simulink model "larix2_tuner_openLoop"  (R2020b)
settings: Solver=FixedStepDiscrete  StartTime=0.0  StopTime=6  FixedStep=0.002  RelTol=1e-3
PostLoadFcn:
  | load('ThrustTable.mat');
  | init();
values from neighbouring files (symbols this model uses):
  eul_0 = [-45*pi/180 0 0]    [init.m]
  g = 9.810    (= 9.81)    [init.m]
  omega_0 = [0 0 0]    [init.m]
  pos_0 = [0 0 0]    [init.m]
  vel_0 = [0 0 0]    [init.m]
undefined symbols (not defined in the file or in its folder): DiscIntNeverNeededParam
libraries: sharedtransform x2
settings Model: Creator=ac114611  LastModifiedBy=wendelin
settings DataIOCC: ExternalInput=getinputstruct(spec2)  InitialState=getstatestruct(spec2)  ReturnWorkspaceOutputs=off
settings OptimizationCC: DefaultParameterBehavior=Inlined  EnhancedBackFolding=on  PassReuseOutputArgsAs=Individual arguments  MaxStackSize=64  OptimizeBlockOrder=speed  DifferentSizesBufferReuse=on  EfficientTunableParamExpr=on
settings DebuggingCC: ParameterPrecisionLossMsg=none  ParameterTunabilityLossMsg=error  ArithmeticOperatorsInVariantConditions=warning
settings HardwareCC: ProdBitPerPointer=32  ProdBitPerSizeT=32  ProdBitPerPtrDiffT=32  ProdLargestAtomicInteger=Long  ProdLargestAtomicFloat=Double  ProdWordSize=32  ProdHWDeviceType=ARM Compatible->ARM Cortex  TargetBitPerLong=64  TargetBitPerPointer=64  TargetBitPerSizeT=64  TargetBitPerPtrDiffT=64  TargetLongLongMode=on  TargetIntDivRoundTo=Zero  TargetEndianess=LittleEndian  TargetWordSize=64  TargetHWDeviceType=MATLAB Host  ProdEqTarget=off
settings SFSimCC: SimUseLocalCustomCode=off  MATLABDynamicMemAlloc=off  CustomCodeUndefinedFunction=UseInterfaceOnly
settings RTWCC: Description=Embedded Coder  SystemTargetFile=ert.tlc  GenCodeOnly=on  PackageName=larix2_codegen.zip  TemplateMakefile=ert_default_tmf  RTWUseLocalCustomCode=off  Toolchain=GNU gcc/g++ | gmake (64-bit Linux)  IncludeHyperlinkInReport=on  GenerateCodeMetricsReport=on
settings CodeAppCC: ForceParamTrailComments=on  IgnoreCustomStorageClasses=off  OperatorAnnotations=on  SimulinkDataObjDesc=on  SFDataObjDesc=on  InsertBlockDesc=on
settings ERTTargetCC: TargetLangStandard=C99 (ISO)  InlinedParameterPlacement=NonHierarchical  ERTCustomFileTemplate=example_file_process.tlc

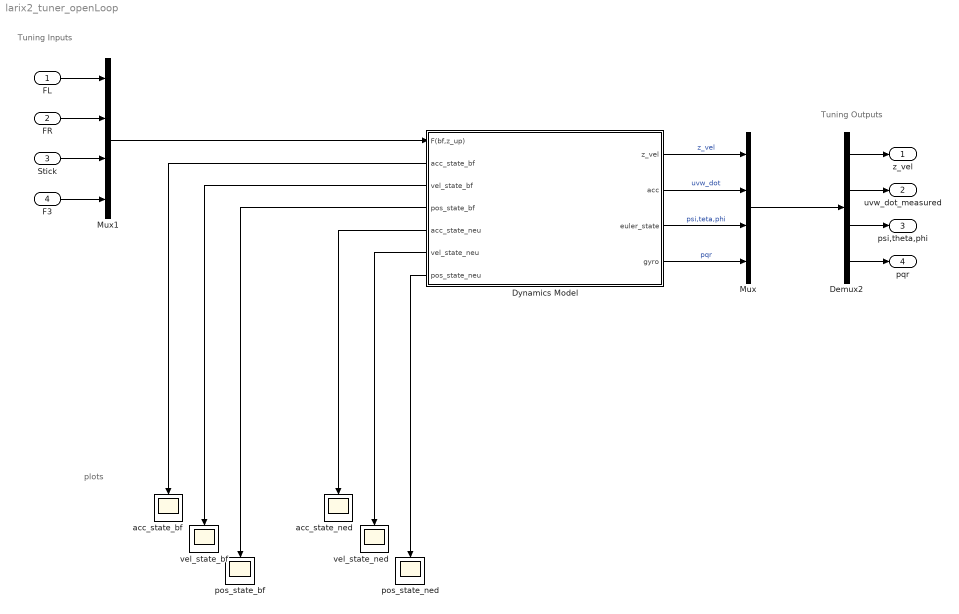
== system larix2_tuner_openLoop ==
  note: Tuning Inputs
  note: Tuning Outputs
  note: plots
  FL : Inport  PortDimensions=1
  FR : Inport  Port=2
  Stick : Inport  Port=3
  F3 : Inport  Port=4
  Demux2 : Demux
  Dynamics Model : Subsystem
      settings: PortSchema="{\"entries\":[{\"content\":{\"sides\":[{\"content\":{\"connectorIds\":[\"In1\",\"Out5\",\"Out6\",\"Out7\",\"Out8\",\"Out9\",\"Out10\"]},\"type\":\"ConnectorPlacement.EquallySpacedRectSide\",\"uuid\":\"7b482eda-451f-4705-a72e-674db1e2ea8f\"},{\"content\":{\"connectorIds\":[\"Out1\",\"Out2\",\"Out3\",\"Out4\"],\"side\":\"RIGHT\"},\"type\":\"ConnectorPlacement.EquallySpacedRectSide\",\"uuid\":\"2344d3e9-2a2c-4bd3-8790-1f9d37abcd4c\"},{\"content\":{\"connectorIds\":[],\"side\":\"TOP\"},\"type\":\"ConnectorPlacement.EquallySpacedRectSide\",\"uuid\":\"13a22bb4-0a82-4477-a366-02f381e5ef07\"},{\"content\":{\"connectorIds\":[],\"side\":\"BOTTOM\"},\"type\":\"ConnectorPlacement.EquallySpacedRectSide\",\"uuid\":\"663825dc-fe4c-484f-87e0-eae3c1c76089\"},{\"content\":{\"connectorIds\":[],\"side\":\"HIDDEN\"},\"type\":\"ConnectorPlacement.EquallySpacedRectSide\",\"uuid\":\"0874c0d1-0ac2-489a-adcf-241d9ac40396\"}]},\"type\":\"ConnectorPlacement.EquallySpacedConnector\",\"uuid\":\"4f633129-49ae-43ab-aa97-bf1abe451306\"}],\"packageUris\":[\"http://schema.mathworks.com/mf0/Connector/R2020b\"],\"version\":\"1.0\"}"
  Mux : Mux
  Mux1 : Mux
  acc_state_bf : Scope
  acc_state_ned : Scope
  pos_state_bf : Scope
  pos_state_ned : Scope
  vel_state_bf : Scope
  vel_state_ned : Scope
  z_vel : Outport  PortDimensions=1
  uvw_dot_measured : Outport  Port=2  PortDimensions=3
  psi,theta,phi : Outport  Port=3  PortDimensions=3
  pqr : Outport  Port=4  PortDimensions=3
  wires:
  Dynamics Model/4(gyro) -> Mux/4  "pqr"
  Dynamics Model/2(acc) -> Mux/2  "uvw_dot"
  Dynamics Model/1(z_vel) -> Mux/1  "z_vel"
  Dynamics Model/3(euler_state) -> Mux/3  "psi,teta,phi"
  Mux/1 -> Demux2/1
  Demux2/1 -> z_vel/1
  Demux2/2 -> uvw_dot_measured/1
  Demux2/4 -> pqr/1
  Demux2/3 -> psi,theta,phi/1
  FL/1 -> Mux1/1
  FR/1 -> Mux1/2
  Stick/1 -> Mux1/3
  F3/1 -> Mux1/4
  Dynamics Model/8(acc_state_neu) -> acc_state_ned/1
  Dynamics Model/6(vel_state_bf) -> vel_state_bf/1
  Dynamics Model/9(vel_state_neu) -> vel_state_ned/1
  Dynamics Model/5(acc_state_bf) -> acc_state_bf/1
  Dynamics Model/7(pos_state_bf) -> pos_state_bf/1
  Dynamics Model/10(pos_state_neu) -> pos_state_ned/1
  Mux1/1 -> Dynamics Model/1(F(bf,z_up))

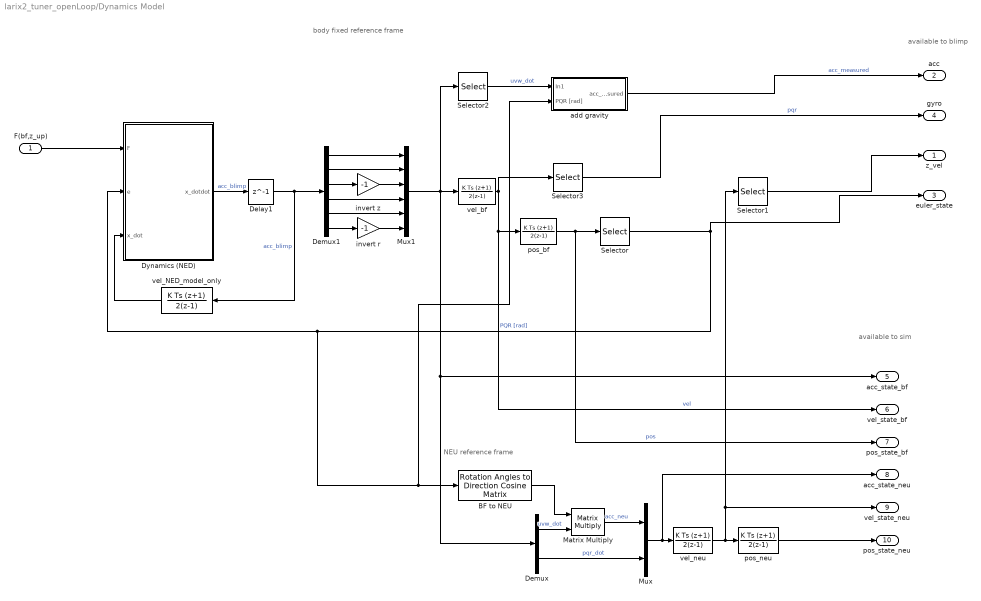
== system larix2_tuner_openLoop/Dynamics Model ==
  note: NEU reference frame
  note: body fixed reference frame
  note: available
      | to sim
  note: available
      | to blimp
  F(bf,z_up) : Inport
  " BF to NEU" : sharedtransform/Rotation Angles to Direction Cosine Matrix  rotationOrder=XYZ  aMode=aMode
      settings: SourceProductBaseCode=AE,PW,MT,UV,VE,VP
  Delay1 : Delay  DelayLength=1  StateName=acc_NED_delay
  Demux : Demux  Outputs=2
  Demux1 : Demux  Outputs=6
  Dynamics (NED) : MATLAB Function  TreatAsAtomicUnit=on
  Matrix Multiply : Product  Multiplication=Matrix(*)
  Mux : Mux  Inputs=2
  Mux1 : Mux  Inputs=6
  Selector : Selector  InputPortWidth=6  IndexOptions=Index vector (dialog)  Indices=[4 5 6]  OutputSizes=1
  Selector1 : Selector  InputPortWidth=6  IndexOptions=Index vector (dialog)  Indices=[3]  OutputSizes=1
  Selector2 : Selector  InputPortWidth=6  IndexOptions=Index vector (dialog)  Indices=[1 2 3]  OutputSizes=1
  Selector3 : Selector  InputPortWidth=6  IndexOptions=Index vector (dialog)  Indices=[4 5 6]  OutputSizes=1
  add gravity : Subsystem
  invert r : Gain  Gain=-1
  invert z : Gain  Gain=-1
  pos_bf : DiscreteIntegrator  IntegratorMethod=Integration: Trapezoidal  InitialCondition=[pos_0,eul_0]  SampleTime=-1  StateName=position_bf  ICPrevOutput=DiscIntNeverNeededParam  ICPrevScaledInput=DiscIntNeverNeededParam
  pos_neu : DiscreteIntegrator  IntegratorMethod=Integration: Trapezoidal  InitialCondition=[pos_0';eul_0']  SampleTime=-1  StateName=position_neu  ICPrevOutput=DiscIntNeverNeededParam  ICPrevScaledInput=DiscIntNeverNeededParam
  vel_NED_model_only : DiscreteIntegrator  IntegratorMethod=Integration: Trapezoidal  SampleTime=-1  StateName=vel_ned  ICPrevOutput=DiscIntNeverNeededParam  ICPrevScaledInput=DiscIntNeverNeededParam
  vel_bf : DiscreteIntegrator  IntegratorMethod=Integration: Trapezoidal  InitialCondition=[vel_0,omega_0]  SampleTime=-1  StateName=velocity_bf  ICPrevOutput=DiscIntNeverNeededParam  ICPrevScaledInput=DiscIntNeverNeededParam
  vel_neu : DiscreteIntegrator  IntegratorMethod=Integration: Trapezoidal  InitialCondition=[pos_0';eul_0']  SampleTime=-1  StateName=velocity_neu  ICPrevOutput=DiscIntNeverNeededParam  ICPrevScaledInput=DiscIntNeverNeededParam
  z_vel : Outport  OutDataTypeStr=double
  acc : Outport  Port=2  OutDataTypeStr=double
  euler_state : Outport  Port=3  OutDataTypeStr=double
  gyro : Outport  Port=4  OutDataTypeStr=double
  acc_state_bf : Outport  Port=5
  vel_state_bf : Outport  Port=6  OutDataTypeStr=double
  pos_state_bf : Outport  Port=7
  acc_state_neu : Outport  Port=8
  vel_state_neu : Outport  Port=9
  pos_state_neu : Outport  Port=10
  wires:
  pos_bf/1 -> pos_state_bf/1, Selector/1  "pos"
  vel_bf/1 -> pos_bf/1, vel_state_bf/1, Selector3/1  "vel"
  F(bf,z_up)/1 -> Dynamics (NED)/1(F)
  Dynamics (NED)/1(x_dotdot) -> Delay1/1  "acc_blimp"
  Selector3/1 -> gyro/1  "pqr"
  pos_neu/1 -> pos_state_neu/1
  Demux/1 -> Matrix Multiply/2  "uvw_dot"
  Demux/2 -> Mux/2  "pqr_dot"
  Matrix Multiply/1 -> Mux/1  "acc_neu"
  Selector/1 -> add gravity/2(PQR [rad]), " BF to NEU"/1, Dynamics (NED)/2(e), euler_state/1  "PQR [rad]"
  " BF to NEU"/1 -> Matrix Multiply/1
  Selector2/1 -> add gravity/1(In1)  "uvw_dot"
  Mux/1 -> acc_state_neu/1, vel_neu/1
  vel_neu/1 -> Selector1/1, vel_state_neu/1, pos_neu/1
  Delay1/1 -> vel_NED_model_only/1, Demux1/1  "acc_blimp"
  Mux1/1 -> Selector2/1, acc_state_bf/1, Demux/1, vel_bf/1
  vel_NED_model_only/1 -> Dynamics (NED)/3(x_dot)
  Demux1/1 -> Mux1/1
  Demux1/2 -> Mux1/2
  Demux1/3 -> invert z/1
  invert z/1 -> Mux1/3
  Demux1/4 -> Mux1/4
  Demux1/5 -> Mux1/5
  Demux1/6 -> invert r/1
  invert r/1 -> Mux1/6
  Selector1/1 -> z_vel/1
  add gravity/1(acc_bf_measured) -> acc/1  "acc_measured"

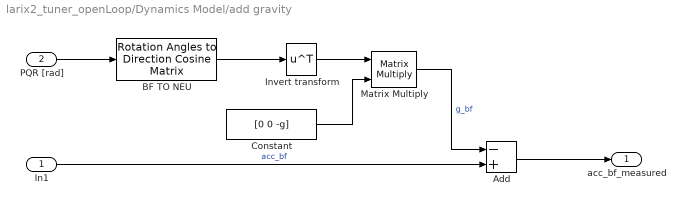
== system larix2_tuner_openLoop/Dynamics Model/add gravity ==
  In1 : Inport
  PQR [rad] : Inport  Port=2
  Add : Sum  Inputs=-+
  BF TO NEU : sharedtransform/Rotation Angles to Direction Cosine Matrix  rotationOrder=XYZ  aMode=aMode
      settings: SourceProductBaseCode=AE,PW,MT,UV,VE,VP
  Constant : Constant  Value=[0 0 -g]
  Invert transform : Math  Operator=transpose  SaturateOnIntegerOverflow=on
  Matrix Multiply : Product  Multiplication=Matrix(*)
  acc_bf_measured : Outport
  wires:
  In1/1 -> Add/2  "acc_bf"
  BF TO NEU/1 -> Invert transform/1
  PQR [rad]/1 -> BF TO NEU/1
  Invert transform/1 -> Matrix Multiply/1
  Matrix Multiply/1 -> Add/1  "g_bf"
  Constant/1 -> Matrix Multiply/2
  Add/1 -> acc_bf_measured/1

== matlab function larix2_tuner_openLoop/Dynamics Model/Dynamics (NED) ==
  data: F input; x_dotdot output; e input; x_dot input
function x_dotdot = fcn(F,e,x_dot)

fL = F(1);
fR = F(2);
stick = F(3);
fB = F(4);

roll = e(1);
pitch = e(2);
yaw = e(3);
%e3 = e(4);


u = x_dot(1);
v = x_dot(2);
w = x_dot(3);
p = x_dot(4);
q = x_dot(5);
r = x_dot(6);

%}

g = 9.81;
rho_air = 1.225; 
eta_air = 1.802e-5;



blimp = inertias();
prp = blimp.prp;
par = blimp.par;
in = blimp.mM;




mx = in.M(1,1);
my = in.M(2,2);
mz = in.M(3,3);

Jxx = in.M(4,4);
Jyy = in.M(5,5);
Jzz = in.M(6,6);
Jxz = in.M(3,6);
 
%DYNAMICS

f1 = -mz*w*q + my*r*v + in.mass*(in.a(1)*( q^2 + r^2) - in.a(3)*r*p);
f2 = -mx*u*r + mz*p*w + in.mass*(-in.a(1)*p*q - in.a(3)*r*q);
f3 = -my*v*p + mx*q*u + in.mass*(-in.a(1)*r*p + in.a(3)*(q^2 + p^2));
f4 = -(Jzz - Jyy)*r*q + Jxz*p*q + in.mass*in.a(3)*(u*r - p*w);
f5 = -(Jxx - Jzz)*p*r + Jxz*(r^2 - p^2) + in.mass*(in.a(1)*(v*p - q*u) - in.a(3)*(w*q - r*v));
f6 = -(Jyy - Jxx)*q*p - Jxz*q*r + in.mass*(-in.a(1)*(u*r - p*w));


F = [f1; f2; f3; f4; f5; f6];

%GRAVITATIONAL FORCES Quaternion
%{
DCM = [e0^2+e1^2-e2^2-e3^2, 2*(e1*e2-e0*e3),2*(e0*e2-e1*e3);...
        2*(e0*e3-e1*e2),e0^2-e1^2+e2^2-e3^2,2*(e2*e3-e0*e1);...
        2*(e1*e3-e0*e2),2*(e0*e1-e2*e3),e0^2-e1^2-e2^2+e3^2];


    
G = [DCM(3,1)*(W+B); DCM(3,2)*(W+B); DCM(3,3)*(W+B);DCM(3,2)*in.a(3)*W; (DCM(3,1)*in.a(3)-DCM(3,3)*in.a(1))*W; DCM(3,2)*in.a(1)*W];
%}



%GRAVITATIONAL FORCES EULER
%{
g_vec = [0 0 g]';

%rot = eul2rotm([e0 e1 e2],'XYZ')';
rot = eul2rotm([roll pitch yaw],'XYZ')';

G_forces = [0 0 h]'*rot*g_vec;

gondola_mass = par.gondola_body.mass + par.gondola_support.mass + par.stick.mass + 2*par.blade_left.mass;      %mass of the whole gondola assembly with its CG at [CG_stick_x 0 CG_stick_z]

G_gondola = gondola_mass*rot*g_vec;


CG_ga = par.stick.position';    %CG coordinates from CV to Gondola assembly

G_moments = cross(G_gondola, CG_ga);

G = [G_forces; G_moments];
%}

h = prp.mass_H;
B = prp.volume_blimp_body*prp.density_air*g;
W = B + h*g;
%%{
rot = eul2rotm([roll pitch yaw],'XYZ');

G = [rot(3,1)*(W-B), rot(3,2)*(W-B), rot(3,3)*(W-B), -rot(3,2)*in.CG(3)*W, (rot(3,1)*in.CG(3) - rot(3,3)*in.CG(1))*W, rot(3,2)*in.CG(1)*W]';
%}
%{
g_vec = [0 0 g];

rotNEDtoBF = eul2rotm([roll pitch yaw],'XYZ');

g_bf = g_vec*rotNEDtoBF;

G = [h*g_bf, cross(in.CG,W*g_bf)]';
%}


%PROPULSION FORCES


rL = blimp.par.blade_left.position';
rR = blimp.par.blade_right.position';
rB = blimp.par.bot_rud_motor.position';

FL = fL*[sin(-stick*pi/2) 0 cos(-stick*pi/2)]';
FR = fR*[sin(-stick*pi/2) 0 cos(-stick*pi/2)]';
FB = fB*[0 1 0]';

TL = cross(rL,FL);
TR = cross(rR,FR);
TB = cross(rB,FB);

Forces = FL+FR+FB;
Torques = TL+TR+TB;

P_NED = [Forces;Torques];

P = P_NED.*[1 1 -1 1 1 -1]';        %convert P from NEU (allocation) to NED 


% AERO FORCES

%AR ~= 0.7 --> nu_fin (Modeling and Simulation of Airship Dynamics)
%finenessratio = 2.375
%hull projected area = 7.461m^2   effective fin area = 0.64 m^2
% effective fin area/ hull projected area = 0.086 --> nu hull

nu_hull =  1.01;
nu_fin = 0.58;

%Cdh0 = 0.3;     %from summary of drag coefficients of various shaped cylinders but reduced because ellipsoid    
Cdh0 = 0.07;    %Theory and Practice of the Hydrodynamic Redesign of Artificial Hellbender Habitat --> closer to value from other papers
Cdf0 = 0.007;    %from Hoerner SF. Fluid Dynamic Drag, Hoerner Fluid Dynamics, 1965. 
Cdg0 = 0.5;     %from Hoerner SF. Fluid Dynamic Drag, Hoerner Fluid Dynamics, 1965. 

Cdhc = 0.5;
Cdfc = 1.2;     %from Hoerner SF. Fluid Dynamic Drag, Hoerner Fluid Dynamics, 1965. 
Cdgc = 0.8;

e = sqrt((prp.length_blimp_a1^2 + prp.radius_blimp_body^2)/prp.length_blimp_a1);

S = pi*prp.radius_blimp_body*(prp.radius_blimp_body+(prp.length_blimp_a1^2)*sin(e)/e);

Vh_ref = prp.volume_blimp_body; %volume based on two semi ellipsoids
Sg_ref = prp.volume_gondola_body^(2/3);
Sh_ref = S;
Sf_ref = 2*prp.surface_two_fins;


fh = (prp.length_tip_to_fin - prp.length_blimp_a1)/prp.length_blimp_a2;
xcv = prp.length_blimp_a1+(3/8)*(prp.length_blimp_a2-prp.length_blimp_a1);
%xcv = prp.length_blimp_a1 - (4*pi/3)*(prp.length_blimp_a1-prp.length_blimp_a2);

I_1 = pi*((prp.radius_blimp_body^2)/Sh_ref)*(1-fh^2);
I_3 = pi*((prp.radius_blimp_body^2)/(3*prp.length_blimp_body*Sh_ref)*(prp.length_blimp_a1 - 2*prp.length_blimp_a2*(fh^3) - 3*prp.length_blimp_a1*(fh^2)) - xcv*I_1/prp.length_blimp_body);


J_1 = prp.radius_blimp_body/(2*Sh_ref)*(pi*prp.length_blimp_a1 + prp.length_blimp_a2*sqrt(1-fh^2)*fh + 2*prp.length_blimp_a2*asin(fh));
J_2 = (J_1/prp.length_blimp_body)*(prp.length_blimp_a1-xcv) + (2*prp.radius_blimp_body/(3*prp.length_blimp_body*Sh_ref))*(prp.length_blimp_a2^2 - prp.length_blimp_a1^2 - (prp.length_blimp_a2^2)*(1-fh^2)^(3/2));

%{
if u == 0
    Cf = 0;
else
Re = abs(u)*prp.length_blimp_body*rho_air/eta_air;
Cf = 0.045*Re^(-1/6);
end

%Cdchull = 1.17;     %Cd of cylinder in transverse flow
%Cdcfin = 1.28;       %Cd of Plate in transverse flow

%Cdcross = -(1/S_ref)*(Cdchull*J_1*S_ref+Cdcfin*S_fin);
%lf1 = 2.35;          %origin to aero/geo center of fin
%lf2 = 2.5;
%}




lf1 = prp.length_tip_to_ac_fin;            %tip to aero center of fin
lf2 = prp.length_tip_to_gc_fin;              %tip to geo center of fin
lf3 = prp.length_yz_origin_to_ac_fin;

U_abs = sqrt(u^2 +v^2 +w^2);


a = atan2(w,u);

if a < 0
    LS = -liftslope(-a);
else
    LS = liftslope(a);
end
    


if U_abs == 0
    b = 0;
else
    b = asin(v/U_abs);
end


%Cx1 = -Cf*(4*(prp.length_blimp_body/prp.radius_blimp_body)^(1/3)+6*(prp.length_blimp_body/prp.radius_blimp_body)^(-1.2)+24*(prp.length_blimp_body/prp.radius_blimp_body)^(-2.7)); %Cd0H        KTh paper       cgcl_xial Cd & b as mcgcl_x_diameter/2 
Cx1 = -(Cdh0*Sh_ref + Cdf0*Sf_ref + Cdg0*Sg_ref);
Cx2 = (in.k(2)-in.k(1))*nu_hull*I_1*Sh_ref;             %munk lift
Cx3 = 0;

Cy1 = -Cx2;                                       
Cy2 = -0.5*LS*Sf_ref*nu_fin;                               %dCl/da = 2*pi  --> only for small angle of attack     from On the lift curve slope for rectangular flat plate wings at moderate Reynolds number
Cy3 = -(Cdhc*J_1*Sh_ref+Cdfc*Sf_ref + Cdgc*Sg_ref);
Cy4 = 0;

Cz1 = -Cx2;
Cz2 = Cy2;
Cz3 = -(Cdhc*J_1*Sh_ref + Cdfc*Sf_ref);       
Cz4 = Cy4;

Cl1 = 0;
Cl2 = Cdgc*Sg_ref*par.gondola_body.position(3);
Cl3 = Cdgc*Sg_ref*par.gondola_body.position(3)*prp.length_blimp_body^2;
Cl4 = -(Cdgc*Sg_ref*par.gondola_body.position(3) + Cdfc*Sf_ref*lf3)*(2*prp.radius_blimp_body)^2;

Cm1 = -(in.k(2)-in.k(1))*nu_hull*I_3*Sh_ref*prp.length_blimp_body;
Cm2 = -0.5*LS*Sf_ref*nu_fin*lf1;
Cm3 = -(Cdhc*J_2*Sh_ref*prp.length_blimp_body + Cdfc*Sf_ref*lf2);
Cm4 = 0;
Cm5 = -Cdfc*Sf_ref*lf2*(prp.length_blimp_body^2);


Cn1 = -Cm1;
Cn2 = -Cm2;
Cn3 = (Cdhc*J_2*Sh_ref*prp.length_blimp_body + Cdfc*Sf_ref*lf2 + Cdgc*Sg_ref*par.gondola_body.position(1));
Cn4 = -Cm4;
Cn5 = -(Cdfc*Sf_ref*lf2 + Cdgc*Sg_ref*par.gondola_body.position(1))*(prp.length_blimp_body^2);

%Cm5 = 0;
%Cn5 = 0;  
    
%e = sqrt(((prp.length_blimp_body*0.5)*(prp.length_blimp_body*0.5)-prp.radius_blimp_body*prp.radius_blimp_body)/(prp.length_blimp_body*0.5));



%{

X = 0.5*rho_air*(U_abs^2)*(Cx1*(cos(a)^2)*(cos(b)^2) + Cx2*sin(2*a)*sin(a/2));
Y = 0.5*rho_air*(U_abs^2)*(Cy1*cos(b/2)*sin(2*b)+Cy2*sin(2*b) + Cy3*sin(b)*sin(abs(b)));
Z = 0.5*rho_air*(U_abs^2)*(Cz1*cos(a/2)*sin(2*a)+Cz2*sin(2*a) + Cz3*sin(a)*sin(abs(a)));

L = 0.5*rho_air*(U_abs^2)*(0.5*rho_air*S*Cl3*p*abs(p));
M = 0.5*rho_air*(U_abs^2)*(Cm1*cos(a/2)*sin(2*a)+Cm2*sin(2*a)+Cm3*sin(a)*sin(abs(a))+0.5*rho_air*S*Cm5*q*abs(q));
N = 0.5*rho_air*(U_abs^2)*(Cn1*cos(b/2)*sin(2*b)+Cn2*sin(2*b)+Cn3*sin(b)*sin(abs(b))+0.5*rho_air*S*Cn5*r*abs(r));

%}

X = 0.5*rho_air*(U_abs^2)*S*(Cx1*(cos(a)^2)*(cos(b)^2) + Cx2*(sin(2*a)*sin(a/2)+sin(2*b)*sin(b/2)+Cx3));
Y = 0.5*rho_air*(U_abs^2)*S*(Cy1*cos(b/2)*sin(2*b)+Cy2*sin(2*b) + Cy3*sin(b)*sin(abs(b)));
Z = 0.5*rho_air*(U_abs^2)*S*(Cz1*cos(a/2)*sin(2*a)+Cz2*sin(2*a) + Cz3*sin(a)*sin(abs(a)));

L = 0.5*rho_air*(U_abs^2)*prp.length_blimp_body*S*(Cl1 + Cl2*(sin(b)*sin(abs(b))) + 0.5*rho_air*S*(Cl3*r*abs(r) + Cl4*p*abs(p)));
M = 0.5*rho_air*(U_abs^2)*prp.length_blimp_body*S*(Cm1*cos(a/2)*sin(2*a) + Cm2*sin(2*a) + Cm3*sin(a)*sin(abs(a)) + Cm4 + 0.5*rho_air*S*Cm5*q*abs(q));
N = 0.5*rho_air*(U_abs^2)*prp.length_blimp_body*S*(Cn1*cos(b/2)*sin(2*b) + Cn2*sin(2*b) + Cn3*sin(b)*sin(abs(b)) + Cn4 + 0.5*rho_air*S*Cn5*r*abs(r));

%Y = 0;
%L = 0;
%N = 0;
 
A = [X;Y;Z;L;M;N];

%masstest = eye(6);
F_sum = (G + A + F + P);

%F_sum(3) = 0;
%F_sum(5) = 0;


%x_dotdot = in.M\(F_sum);
x_dotdot = in.M_inv*(F_sum);
end
